simulink model "LACS"  (R2016b)
settings: Solver=VariableStepAuto  StartTime=0.0  StopTime=10  RelTol=1e-3
values from neighbouring files (symbols this model uses):
  coefficient = 0.8    [LACS.sldd]
  Detal_ref = 0.00022116955850615819 0.00022116955850615819 0.00024339323736781077 0.00026784369743330114 0.00029474273075037104 0.00032433393975435165 0.00035688482250496254 0.00039268904453642435 0.00043206891122917146 0.00047537805500027884 0.00052300435183202216 0.00057537308165349073 0.00063295034678974044 0.00069624676200566427 0.00076582142849131239 0.0008422862023284908 0.000926310265386283 0.0010186250    [LACS.sldd]    (also in path_generate.m = zeros(N,1))
  driver_decel = 4.0    [LACS.sldd]
  EgoLength = 3.048    [LACS.sldd]
  egopath = 0.0 0.25 0.5 0.75 1.0 1.25 1.5 1.7500000000000002 2.0 2.25 2.5 2.75 3.0 3.25 3.5000000000000004 3.75 4.0 4.25 4.5 4.75 5.0 5.25 5.5 5.75 6.0 6.25 6.5 6.75 7.0000000000000009 7.2499999999999991 7.5 7.75 8.0 8.25 8.5 8.75 9.0 9.25 9.5 9.75 10.0 10.25 10.5 10.75 11.0 11.25 11.5 11.75 12.0 12.25 12.5 12.75 13.0 13.25 13.5 13.750000000000002 14.000000000000002 14.250000000000002 14.499999999999998 14.7    [LACS.sldd]
  egoSpdLimit_H = 150.0    [LACS.sldd]
  egoSpdLimit_L = 10.0    [LACS.sldd]
  EgoWidth = 1.628    [LACS.sldd]
  ESA_Active = 3.0    [LACS.sldd]
  ESA_mask_1 = 31.0    [LACS.sldd]
  ESA_mask_2 = 15.0    [LACS.sldd]
  ESA_mask_3 = 255.0    [LACS.sldd]
  ESA_mask_4 = 31.0    [LACS.sldd]
  ESA_Passive = 1.0    [LACS.sldd]
  ESA_Standby = 2.0    [LACS.sldd]
  g = 9.8    [LACS.sldd]
  headwayoffset = 1.524    [LACS.sldd]
  LatAccelThershold = 0.05    [LACS.sldd]
  LatDis = 0.5    [LACS.sldd]
  LatSafetyThershold = 0.5    [LACS.sldd]
  LengthObj = 3.0    [LACS.sldd]
  ObjWidth = 2.0    [LACS.sldd]
  PB1_decel = 3.0    [LACS.sldd]
  PB2_decel = 5.0    [LACS.sldd]
  PB3_decel = 8.0    [LACS.sldd]
  Phi_dot_ref = 0.00085065224568106894 0.00085065224568106894 0.000936127966106986 0.0010301682404378703 0.0011336261186052523 0.0012474385378394444 0.001372634343205976 0.0015103430260158721 0.001661804233646022 0.0018283781058153412 0.0020115564932359636 0.0022129751145658549 0.0024344267064660809 0.0026778752189651235 0.0029454711038487576 0.0032395677369184911 0.0035627390050890382 0.0039177980756855638 0.004    [LACS.sldd]    (also in path_generate.m = zeros(N,1))
  Phi_ref = 0.00038406250525431664 0.00042271073336932769 0.00046524334565338114 0.00051204974395873044 0.000563558155980624 0.00062023946191088657 0.00068261138880285879 0.00075124310596315759 0.0008267602572639512 0.0009098504689462523 0.0010012693742370194 0.0011018471988988175 0.0012124959546271103 0.0013342172899504143 0.0014681110508986705 0.0016153846060911084 0.0017773629929370329 0.001955499943191484    [LACS.sldd]    (also in path_generate.m = phi_ref)
  SteerAngleLimit = 20.0    [LACS.sldd]
  SteerAngleSpdLimit = 20.0    [LACS.sldd]
  StrAngSpdThershold = 0.05    [LACS.sldd]
  StrAngThershold = 0.0    [LACS.sldd]
  Time2React = 1.2    [LACS.sldd]
  timeMargin = 0.5    [LACS.sldd]
  TTCthreshold1 = 2.5    [LACS.sldd]
  TTCthreshold3 = 1.0    [LACS.sldd]
  X_dot_ref = 10.0 10.0 10.0 9.9999999999999947 10.0 10.0 10.0 10.0 10.0 10.0 10.0 10.0 10.0 10.0 10.0 10.000000000000018 10.0 10.0 10.0 10.0 10.0 10.0 10.0 10.0 10.0 10.0 10.0 10.0 10.0 10.0 10.0 10.0 10.0 10.0 10.0 10.0 10.0 10.0 10.0 10.0 10.0 10.0 10.0 10.0 10.0 10.0 10.0 10.0 10.0 10.0 10.0 10.0 10.0 10.0 10.0 10.0 10.0 10.0 10.0 10.0 10.0 10.0 10.0 9.9999999999999289 10.0 10.0 10.0 10.0 10.0 10.0 10.0 10.    [LACS.sldd]    (also in path_generate.m = zeros(N,1))
  X_ref = 0.05 0.55 1.05 1.55 2.05 2.55 3.05 3.55 4.05 4.55 5.05 5.55 6.05 6.55 7.05 7.55 8.05 8.55 9.05 9.55 10.05 10.55 11.05 11.55 12.05 12.55 13.05 13.55 14.05 14.55 15.05 15.55 16.05 16.55 17.05 17.55 18.05 18.55 19.05 19.55 20.05 20.55 21.05 21.55 22.05 22.55 23.05 23.55 24.05 24.55 25.05 25.55 26.05 26.55 27.05 27.55 28.05 28.55 29.05 29.55 30.05 30.55 31.05 31.55 32.05 32.55 33.05 33.55 34.05 34.55    [LACS.sldd]    (also in path_generate.m = X_phi')
  Y_dot_ref = 0.0044363771042237217 0.0044363771042237217 0.00488273213335339 0.0053739322979981 0.0059144698111347933 0.0065092840662692251 0.0071638055584438178 0.0078840039934084845 0.0086764409570179273 0.0095483275445279979 0.01050758737719603 0.011562925461771293 0.012723903376023141 0.014001021290828194 0.015405807364013962 0.016950915064438028 0.018650229002128878 0.020518979854070446 0.0225738689793052    [LACS.sldd]    (also in path_generate.m = zeros(N,1))
  Y_ref = 0.0020016327462461514 0.0022031718511841521 0.0024249907063953382 0.0026691273130630077 0.0029378239279629127 0.0032335474185196523 0.0035590116218331136 0.0039172018997553045 0.0043114020994257287 0.0047452241472766251 0.005222640524503025 0.0057480198933628265 0.0063261661664513911 0.0069623613352525482 0.0076624123997939579 0.008432702767994656 0.0092802485212165574 0.010212759971323001 0.01123    [LACS.sldd]    (also in path_generate.m = zeros(N,1))
undefined symbols (not defined in the file or in its folder): ADR_ADRCycleTime, ADR_SteeringYawrateThresh_p, AEB_mask1, aubr, CAEB_AccelPdlPosLimit, CAEB_AccelPdlPosSpdThreshold, CAEB_CalAEBLongVelObjLimit_mps, CAEB_CalAEBVMaxDec_kmph, ESA_AESACTIVE, ESA_ERROR, ESA_ESAFunctionOFF, ESA_ESAFunctionON, ESA_ESASwichOFF, ESA_ESS_DriverSteeringNumThreshold, ESA_ESSACTIVE, ESA_ForewardCollissionLevel2, ESA_ForewardCollissionLevel3, ESA_OFF, ESA_PASSIVE, ESA_PLAN_AES, ESA_PLAN_ESSLEFT, ESA_PLAN_ESSRIGHT, ESA_PLAN_FAILURE, ESA_PLAN_OFF, ESA_PLAN_STANDBY, ESA_PLAN_WAIT, ESA_SPEEDLIMITH6_p, ESA_SPEEDLIMITH7_p, ESA_SPEEDLIMITL6_p, ESA_SPEEDLIMITL7_p, ESA_STANDBY, ESA_StrAngSpdT6_p, FromAngle2Rad, Kp, magnitude, tablebr, TTCthreshold, vubr
libraries: simulink x15, Solver_SF x9, simulink_extras x1
(part 4 of 5)

== system LACS/ESAsts/Passive2StandbyFlag/Subsystem3 ==
  flag : Inport
  Constant45 : Constant  Value=0  OutDataTypeStr=uint32
  Constant46 : Constant  OutDataTypeStr=uint32
  Multiport Switch7 : MultiPortSwitch  DataPortOrder=Zero-based contiguous  Inputs=2
  Shift Arithmetic : ArithShift  BitShiftNumberSource=Input port  BitShiftNumber=8  BitShiftDirection=Left
      settings: InputPortMap=u0,p1
  bitMask : Constant  Value=0  OutDataTypeStr=uint8
  maskCnst : Outport
  wires:
  flag/1 -> Multiport Switch7/1
  Multiport Switch7/1 -> maskCnst/1
  Constant46/1 -> Shift Arithmetic/1
  Constant45/1 -> Multiport Switch7/2
  Shift Arithmetic/1 -> Multiport Switch7/3
  bitMask/1 -> Shift Arithmetic/2

== system LACS/ESAsts/Passive2StandbyFlag/Subsystem4 ==
  flag : Inport
  Constant45 : Constant  Value=0  OutDataTypeStr=uint32
  Constant46 : Constant  OutDataTypeStr=uint32
  Multiport Switch7 : MultiPortSwitch  DataPortOrder=Zero-based contiguous  Inputs=2
  Shift Arithmetic : ArithShift  BitShiftNumberSource=Input port  BitShiftNumber=8  BitShiftDirection=Left
      settings: InputPortMap=u0,p1
  bitMask : Constant  Value=2  OutDataTypeStr=uint8
  maskCnst : Outport
  wires:
  flag/1 -> Multiport Switch7/1
  Multiport Switch7/1 -> maskCnst/1
  Constant46/1 -> Shift Arithmetic/1
  Constant45/1 -> Multiport Switch7/2
  Shift Arithmetic/1 -> Multiport Switch7/3
  bitMask/1 -> Shift Arithmetic/2

== system LACS/ESAsts/Passive2StandbyFlag/Subsystem5 ==
  flag : Inport
  Constant45 : Constant  Value=0  OutDataTypeStr=uint32
  Constant46 : Constant  OutDataTypeStr=uint32
  Multiport Switch7 : MultiPortSwitch  DataPortOrder=Zero-based contiguous  Inputs=2
  Shift Arithmetic : ArithShift  BitShiftNumberSource=Input port  BitShiftNumber=8  BitShiftDirection=Left
      settings: InputPortMap=u0,p1
  bitMask : Constant  Value=3  OutDataTypeStr=uint8
  maskCnst : Outport
  wires:
  flag/1 -> Multiport Switch7/1
  Multiport Switch7/1 -> maskCnst/1
  Constant46/1 -> Shift Arithmetic/1
  Constant45/1 -> Multiport Switch7/2
  Shift Arithmetic/1 -> Multiport Switch7/3
  bitMask/1 -> Shift Arithmetic/2

== system LACS/ESAsts/Passive2StandbyFlag1/LatAccelLimit ==
  Constant10 : Constant  Value=g
  Constant12 : Constant  Value=0.67
  Constant9 : Constant  Value=coefficient
  Divide : Product  Inputs=***
  Limit : Outport
  wires:
  Constant10/1 -> Divide/2
  Constant12/1 -> Divide/3
  Divide/1 -> Limit/1
  Constant9/1 -> Divide/1

== system LACS/ESAsts/Passive2StandbyFlag1/Subsystem1 ==
  flag : Inport
  Constant45 : Constant  Value=0  OutDataTypeStr=uint32
  Constant46 : Constant  OutDataTypeStr=uint32
  Multiport Switch7 : MultiPortSwitch  DataPortOrder=Zero-based contiguous  Inputs=2
  Shift Arithmetic : ArithShift  BitShiftNumberSource=Input port  BitShiftNumber=8  BitShiftDirection=Left
      settings: InputPortMap=u0,p1
  bitMask : Constant  Value=0  OutDataTypeStr=uint8
  maskCnst : Outport
  wires:
  flag/1 -> Multiport Switch7/1
  Multiport Switch7/1 -> maskCnst/1
  Constant46/1 -> Shift Arithmetic/1
  Constant45/1 -> Multiport Switch7/2
  Shift Arithmetic/1 -> Multiport Switch7/3
  bitMask/1 -> Shift Arithmetic/2

== system LACS/ESAsts/Passive2StandbyFlag1/Subsystem16 ==
  flag : Inport
  Constant45 : Constant  Value=0  OutDataTypeStr=uint32
  Constant46 : Constant  Value=2  OutDataTypeStr=uint32
  Multiport Switch7 : MultiPortSwitch  DataPortOrder=Zero-based contiguous  Inputs=2
  Shift Arithmetic : ArithShift  BitShiftNumberSource=Input port  BitShiftNumber=8  BitShiftDirection=Left
      settings: InputPortMap=u0,p1
  bitMask : Constant  Value=0  OutDataTypeStr=uint8
  maskCnst : Outport
  wires:
  flag/1 -> Multiport Switch7/1
  Multiport Switch7/1 -> maskCnst/1
  Constant46/1 -> Shift Arithmetic/1
  Constant45/1 -> Multiport Switch7/2
  Shift Arithmetic/1 -> Multiport Switch7/3
  bitMask/1 -> Shift Arithmetic/2

== system LACS/ESAsts/Passive2StandbyFlag1/Subsystem2 ==
  flag : Inport
  Constant45 : Constant  Value=0  OutDataTypeStr=uint32
  Constant46 : Constant  Value=3  OutDataTypeStr=uint32
  Multiport Switch7 : MultiPortSwitch  DataPortOrder=Zero-based contiguous  Inputs=2
  Shift Arithmetic : ArithShift  BitShiftNumberSource=Input port  BitShiftNumber=8  BitShiftDirection=Left
      settings: InputPortMap=u0,p1
  bitMask : Constant  Value=0  OutDataTypeStr=uint8
  maskCnst : Outport
  wires:
  bitMask/1 -> Shift Arithmetic/2
  Shift Arithmetic/1 -> Multiport Switch7/3
  Constant45/1 -> Multiport Switch7/2
  Constant46/1 -> Shift Arithmetic/1
  Multiport Switch7/1 -> maskCnst/1
  flag/1 -> Multiport Switch7/1

== system LACS/ESAsts/Passive2StandbyFlag1/Subsystem3 ==
  flag : Inport
  Constant45 : Constant  Value=0  OutDataTypeStr=uint32
  Constant46 : Constant  Value=4  OutDataTypeStr=uint32
  Multiport Switch7 : MultiPortSwitch  DataPortOrder=Zero-based contiguous  Inputs=2
  Shift Arithmetic : ArithShift  BitShiftNumberSource=Input port  BitShiftNumber=8  BitShiftDirection=Left
      settings: InputPortMap=u0,p1
  bitMask : Constant  Value=0  OutDataTypeStr=uint8
  maskCnst : Outport
  wires:
  bitMask/1 -> Shift Arithmetic/2
  Shift Arithmetic/1 -> Multiport Switch7/3
  Constant45/1 -> Multiport Switch7/2
  Constant46/1 -> Shift Arithmetic/1
  Multiport Switch7/1 -> maskCnst/1
  flag/1 -> Multiport Switch7/1

== system LACS/ESAsts/Passive2StandbyFlag1/Subsystem4 ==
  flag : Inport
  Constant45 : Constant  Value=0  OutDataTypeStr=uint32
  Constant46 : Constant  Value=5  OutDataTypeStr=uint32
  Multiport Switch7 : MultiPortSwitch  DataPortOrder=Zero-based contiguous  Inputs=2
  Shift Arithmetic : ArithShift  BitShiftNumberSource=Input port  BitShiftNumber=8  BitShiftDirection=Left
      settings: InputPortMap=u0,p1
  bitMask : Constant  Value=0  OutDataTypeStr=uint8
  maskCnst : Outport
  wires:
  flag/1 -> Multiport Switch7/1
  Multiport Switch7/1 -> maskCnst/1
  Constant46/1 -> Shift Arithmetic/1
  Constant45/1 -> Multiport Switch7/2
  Shift Arithmetic/1 -> Multiport Switch7/3
  bitMask/1 -> Shift Arithmetic/2

== system LACS/ESAsts/Passive2StandbyFlag1/Subsystem5 ==
  flag : Inport
  Constant45 : Constant  Value=0  OutDataTypeStr=uint32
  Constant46 : Constant  Value=6  OutDataTypeStr=uint32
  Multiport Switch7 : MultiPortSwitch  DataPortOrder=Zero-based contiguous  Inputs=2
  Shift Arithmetic : ArithShift  BitShiftNumberSource=Input port  BitShiftNumber=8  BitShiftDirection=Left
      settings: InputPortMap=u0,p1
  bitMask : Constant  Value=0  OutDataTypeStr=uint8
  maskCnst : Outport
  wires:
  flag/1 -> Multiport Switch7/1
  Multiport Switch7/1 -> maskCnst/1
  Constant46/1 -> Shift Arithmetic/1
  Constant45/1 -> Multiport Switch7/2
  Shift Arithmetic/1 -> Multiport Switch7/3
  bitMask/1 -> Shift Arithmetic/2

== system LACS/ESAsts/Stanby2PassiveFlag/LatAccelLimit ==
  Constant10 : Constant  Value=g
  Constant12 : Constant  Value=0.67
  Constant9 : Constant  Value=coefficient
  Divide : Product  Inputs=***
  Limit : Outport
  wires:
  Constant10/1 -> Divide/2
  Constant12/1 -> Divide/3
  Divide/1 -> Limit/1
  Constant9/1 -> Divide/1

== system LACS/ESAsts/Stanby2PassiveFlag/Subsystem1 ==
  flag : Inport
  Constant45 : Constant  Value=0  OutDataTypeStr=uint32
  Constant46 : Constant  OutDataTypeStr=uint32
  Multiport Switch7 : MultiPortSwitch  DataPortOrder=Zero-based contiguous  Inputs=2
  Shift Arithmetic : ArithShift  BitShiftNumberSource=Input port  BitShiftNumber=8  BitShiftDirection=Left
      settings: InputPortMap=u0,p1
  bitMask : Constant  Value=3  OutDataTypeStr=uint8
  maskCnst : Outport
  wires:
  flag/1 -> Multiport Switch7/1
  Multiport Switch7/1 -> maskCnst/1
  Constant46/1 -> Shift Arithmetic/1
  Constant45/1 -> Multiport Switch7/2
  Shift Arithmetic/1 -> Multiport Switch7/3
  bitMask/1 -> Shift Arithmetic/2

== system LACS/ESAsts/Stanby2PassiveFlag/Subsystem3 ==
  flag : Inport
  Constant45 : Constant  Value=0  OutDataTypeStr=uint32
  Constant46 : Constant  OutDataTypeStr=uint32
  Multiport Switch7 : MultiPortSwitch  DataPortOrder=Zero-based contiguous  Inputs=2
  Shift Arithmetic : ArithShift  BitShiftNumberSource=Input port  BitShiftNumber=8  BitShiftDirection=Left
      settings: InputPortMap=u0,p1
  bitMask : Constant  Value=0  OutDataTypeStr=uint8
  maskCnst : Outport
  wires:
  flag/1 -> Multiport Switch7/1
  Multiport Switch7/1 -> maskCnst/1
  Constant46/1 -> Shift Arithmetic/1
  Constant45/1 -> Multiport Switch7/2
  Shift Arithmetic/1 -> Multiport Switch7/3
  bitMask/1 -> Shift Arithmetic/2

== system LACS/ESAsts/Stanby2PassiveFlag/Subsystem4 ==
  flag : Inport
  Constant45 : Constant  Value=0  OutDataTypeStr=uint32
  Constant46 : Constant  OutDataTypeStr=uint32
  Multiport Switch7 : MultiPortSwitch  DataPortOrder=Zero-based contiguous  Inputs=2
  Shift Arithmetic : ArithShift  BitShiftNumberSource=Input port  BitShiftNumber=8  BitShiftDirection=Left
      settings: InputPortMap=u0,p1
  bitMask : Constant  OutDataTypeStr=uint8
  maskCnst : Outport
  wires:
  flag/1 -> Multiport Switch7/1
  Multiport Switch7/1 -> maskCnst/1
  Constant46/1 -> Shift Arithmetic/1
  Constant45/1 -> Multiport Switch7/2
  Shift Arithmetic/1 -> Multiport Switch7/3
  bitMask/1 -> Shift Arithmetic/2

== system LACS/ESAsts/Stanby2PassiveFlag/Subsystem5 ==
  flag : Inport
  Constant45 : Constant  Value=0  OutDataTypeStr=uint32
  Constant46 : Constant  OutDataTypeStr=uint32
  Multiport Switch7 : MultiPortSwitch  DataPortOrder=Zero-based contiguous  Inputs=2
  Shift Arithmetic : ArithShift  BitShiftNumberSource=Input port  BitShiftNumber=8  BitShiftDirection=Left
      settings: InputPortMap=u0,p1
  bitMask : Constant  Value=2  OutDataTypeStr=uint8
  maskCnst : Outport
  wires:
  flag/1 -> Multiport Switch7/1
  Multiport Switch7/1 -> maskCnst/1
  Constant46/1 -> Shift Arithmetic/1
  Constant45/1 -> Multiport Switch7/2
  Shift Arithmetic/1 -> Multiport Switch7/3
  bitMask/1 -> Shift Arithmetic/2

== system LACS/ESAsts/Standby to Active/LatAccelLimit ==
  Constant10 : Constant  Value=g
  Constant12 : Constant  Value=0.67
  Constant9 : Constant  Value=coefficient
  Divide : Product  Inputs=***
  Limit : Outport
  wires:
  Constant10/1 -> Divide/2
  Constant12/1 -> Divide/3
  Divide/1 -> Limit/1
  Constant9/1 -> Divide/1

== system LACS/ESAsts/Standby to Active/Subsystem1 ==
  flag : Inport
  Constant45 : Constant  Value=0  OutDataTypeStr=uint32
  Constant46 : Constant  OutDataTypeStr=uint32
  Multiport Switch7 : MultiPortSwitch  DataPortOrder=Zero-based contiguous  Inputs=2
  Shift Arithmetic : ArithShift  BitShiftNumberSource=Input port  BitShiftNumber=8  BitShiftDirection=Left
      settings: InputPortMap=u0,p1
  bitMask : Constant  OutDataTypeStr=uint8
  maskCnst : Outport
  wires:
  flag/1 -> Multiport Switch7/1
  Multiport Switch7/1 -> maskCnst/1
  Constant46/1 -> Shift Arithmetic/1
  Constant45/1 -> Multiport Switch7/2
  Shift Arithmetic/1 -> Multiport Switch7/3
  bitMask/1 -> Shift Arithmetic/2

== system LACS/ESAsts/Standby to Active/Subsystem16 ==
  flag : Inport
  Constant45 : Constant  Value=0  OutDataTypeStr=uint32
  Constant46 : Constant  OutDataTypeStr=uint32
  Multiport Switch7 : MultiPortSwitch  DataPortOrder=Zero-based contiguous  Inputs=2
  Shift Arithmetic : ArithShift  BitShiftNumberSource=Input port  BitShiftNumber=8  BitShiftDirection=Left
      settings: InputPortMap=u0,p1
  bitMask : Constant  Value=2  OutDataTypeStr=uint8
  maskCnst : Outport
  wires:
  flag/1 -> Multiport Switch7/1
  Multiport Switch7/1 -> maskCnst/1
  Constant46/1 -> Shift Arithmetic/1
  Constant45/1 -> Multiport Switch7/2
  Shift Arithmetic/1 -> Multiport Switch7/3
  bitMask/1 -> Shift Arithmetic/2

== system LACS/ESAsts/Standby to Active/Subsystem2 ==
  flag : Inport
  Constant45 : Constant  Value=0  OutDataTypeStr=uint32
  Constant46 : Constant  OutDataTypeStr=uint32
  Multiport Switch7 : MultiPortSwitch  DataPortOrder=Zero-based contiguous  Inputs=2
  Shift Arithmetic : ArithShift  BitShiftNumberSource=Input port  BitShiftNumber=8  BitShiftDirection=Left
      settings: InputPortMap=u0,p1
  bitMask : Constant  Value=3  OutDataTypeStr=uint8
  maskCnst : Outport
  wires:
  bitMask/1 -> Shift Arithmetic/2
  Shift Arithmetic/1 -> Multiport Switch7/3
  Constant45/1 -> Multiport Switch7/2
  Constant46/1 -> Shift Arithmetic/1
  Multiport Switch7/1 -> maskCnst/1
  flag/1 -> Multiport Switch7/1

== system LACS/ESAsts/Standby to Active/Subsystem3 ==
  flag : Inport
  Constant45 : Constant  Value=0  OutDataTypeStr=uint32
  Constant46 : Constant  OutDataTypeStr=uint32
  Multiport Switch7 : MultiPortSwitch  DataPortOrder=Zero-based contiguous  Inputs=2
  Shift Arithmetic : ArithShift  BitShiftNumberSource=Input port  BitShiftNumber=8  BitShiftDirection=Left
      settings: InputPortMap=u0,p1
  bitMask : Constant  Value=4  OutDataTypeStr=uint8
  maskCnst : Outport
  wires:
  bitMask/1 -> Shift Arithmetic/2
  Shift Arithmetic/1 -> Multiport Switch7/3
  Constant45/1 -> Multiport Switch7/2
  Constant46/1 -> Shift Arithmetic/1
  Multiport Switch7/1 -> maskCnst/1
  flag/1 -> Multiport Switch7/1

== system LACS/ESAsts/Standby to Active/Subsystem4 ==
  flag : Inport
  Constant45 : Constant  Value=0  OutDataTypeStr=uint32
  Constant46 : Constant  OutDataTypeStr=uint32
  Multiport Switch7 : MultiPortSwitch  DataPortOrder=Zero-based contiguous  Inputs=2
  Shift Arithmetic : ArithShift  BitShiftNumberSource=Input port  BitShiftNumber=8  BitShiftDirection=Left
      settings: InputPortMap=u0,p1
  bitMask : Constant  Value=5  OutDataTypeStr=uint8
  maskCnst : Outport
  wires:
  flag/1 -> Multiport Switch7/1
  Multiport Switch7/1 -> maskCnst/1
  Constant46/1 -> Shift Arithmetic/1
  Constant45/1 -> Multiport Switch7/2
  Shift Arithmetic/1 -> Multiport Switch7/3
  bitMask/1 -> Shift Arithmetic/2

== system LACS/ESAsts/Standby to Active/Subsystem5 ==
  flag : Inport
  Constant45 : Constant  Value=0  OutDataTypeStr=uint32
  Constant46 : Constant  OutDataTypeStr=uint32
  Multiport Switch7 : MultiPortSwitch  DataPortOrder=Zero-based contiguous  Inputs=2
  Shift Arithmetic : ArithShift  BitShiftNumberSource=Input port  BitShiftNumber=8  BitShiftDirection=Left
      settings: InputPortMap=u0,p1
  bitMask : Constant  Value=6  OutDataTypeStr=uint8
  maskCnst : Outport
  wires:
  flag/1 -> Multiport Switch7/1
  Multiport Switch7/1 -> maskCnst/1
  Constant46/1 -> Shift Arithmetic/1
  Constant45/1 -> Multiport Switch7/2
  Shift Arithmetic/1 -> Multiport Switch7/3
  bitMask/1 -> Shift Arithmetic/2

== system LACS/ESAsts/Standby to Active/Subsystem6 ==
  flag : Inport
  Constant45 : Constant  Value=0  OutDataTypeStr=uint32
  Constant46 : Constant  OutDataTypeStr=uint32
  Multiport Switch7 : MultiPortSwitch  DataPortOrder=Zero-based contiguous  Inputs=2
  Shift Arithmetic : ArithShift  BitShiftNumberSource=Input port  BitShiftNumber=8  BitShiftDirection=Left
      settings: InputPortMap=u0,p1
  bitMask : Constant  Value=0  OutDataTypeStr=uint8
  maskCnst : Outport
  wires:
  flag/1 -> Multiport Switch7/1
  Multiport Switch7/1 -> maskCnst/1
  Constant46/1 -> Shift Arithmetic/1
  Constant45/1 -> Multiport Switch7/2
  Shift Arithmetic/1 -> Multiport Switch7/3
  bitMask/1 -> Shift Arithmetic/2

== system LACS/ESAsts/Standby to Active/Subsystem7 ==
  flag : Inport
  Constant45 : Constant  Value=0  OutDataTypeStr=uint32
  Constant46 : Constant  OutDataTypeStr=uint32
  Multiport Switch7 : MultiPortSwitch  DataPortOrder=Zero-based contiguous  Inputs=2
  Shift Arithmetic : ArithShift  BitShiftNumberSource=Input port  BitShiftNumber=8  BitShiftDirection=Left
      settings: InputPortMap=u0,p1
  bitMask : Constant  Value=7  OutDataTypeStr=uint8
  maskCnst : Outport
  wires:
  flag/1 -> Multiport Switch7/1
  Multiport Switch7/1 -> maskCnst/1
  Constant46/1 -> Shift Arithmetic/1
  Constant45/1 -> Multiport Switch7/2
  Shift Arithmetic/1 -> Multiport Switch7/3
  bitMask/1 -> Shift Arithmetic/2

== stateflow chart LACS/ESAManager ==
  state ON
    FuncStsReq = ESA_ESAFunctionON;
    state STANDBY
      en, du:
      EsaSts = ESA_STANDBY;
      EsaSts_plan = ESA_PLAN_WAIT;
      TakeoverFbk = false;
    state PASSIVE
      en, du:
      EsaSts = ESA_PASSIVE;
      EsaSts_plan = ESA_PLAN_STANDBY;
      TakeoverFbk = false;
    state ACTIVE
      TakeoverFbk = true;
      state ESSACTIVE
        en, du:
        EsaSts = ESA_ESSACTIVE;
        state ESSRIGHT
          en, du:
          EsaSts_plan = ESA_PLAN_ESSRIGHT;
        state ESSLEFT
          en, du:
          EsaSts_plan = ESA_PLAN_ESSLEFT;
      state ASSACTIVE
        en, du:
        EsaSts = ESA_AESACTIVE;
        EsaSts_plan = ESA_PLAN_AES;
    (default) -> PASSIVE
    PASSIVE -> STANDBY : /*C4*/
        | after(1, tick)
        | [fc4]
    STANDBY -> PASSIVE [order 3] : /*C5*/
        | after(1, tick)
        | [fc5]
    ACTIVE -> PASSIVE : /*C8*/
        | after(1, tick)
        | [fc8]
    STANDBY -> ESSLEFT [order 1] : /*C6*/
        | after(1, tick)
        | [fc6_left]
    STANDBY -> ESSRIGHT [order 4] : after(1, tick)
        | [fc6_right]
    STANDBY -> ASSACTIVE [order 2] : /*C7*/
        | after(1, tick)
        | [fc7]
  state OFF
    en, du:
    EsaSts = ESA_OFF;
    EsaSts_plan = ESA_PLAN_OFF;
    TakeoverFbk = false;
    FuncStsReq = ESA_ESAFunctionOFF;
  state ERROR
    en, du:
    EsaSts = ESA_ERROR;
    EsaSts_plan = ESA_PLAN_FAILURE;
    TakeoverFbk = false;
    FuncStsReq = ESA_ESAFunctionOFF;
  (default) -> ON
  OFF -> ON : /**C1*/
      | after(1, tick)
      | [fc1]
  ON -> OFF [order 1] : /*C2**/
      | after(1, tick)
      | [fc2]
  ERROR -> ON : /*C10*/
      | after(1, tick)
      | [fc10]
  ON -> ERROR [order 2] : /*C9*/
      | after(1, tick)
      | [fc9]
  data: fc1 input boolean; fc2 input boolean; ESA_AESACTIVE parameter uint8; ESA_ERROR parameter uint8; ESA_ESSACTIVE parameter uint8; ESA_OFF parameter uint8; ESA_PASSIVE parameter uint8; ESA_STANDBY parameter uint8; EsaSts output uint8; fc4 input boolean; fc5 input boolean; fc6_left input boolean; fc6_right input boolean; fc7 input boolean; fc8 input boolean; fc9 input boolean; fc10 input boolean; FuncStsReq output uint8; TakeoverFbk output boolean; EsaSts_plan output uint8; ESA_PLAN_AES parameter; ESA_PLAN_ESSLEFT parameter; ESA_PLAN_ESSRIGHT parameter; ESA_PLAN_FAILURE parameter; ESA_PLAN_OFF parameter; ESA_PLAN_STANDBY parameter; ESA_PLAN_WAIT parameter; ESA_ESAFunctionOFF parameter uint8; ESA_ESAFunctionON parameter uint8

== stateflow chart LACS/AEB_System/Chart ==
  state default_state
    entry:CMpa = 0;
    Alart = 0;
    Break_signal = 0;
  state Init_1_state1
    du:
    if(30<Distance<40)
    CMpa = 2;
    Alart = 1;
    Break_signal = 1;
    elseif(20<Distance<30)
    CMpa = 5;
    Alart = 2;
    Break_signal = 1;
    elseif(10<Distance<20)
    CMpa = 8;
    Alart = 3;
    Break_signal = 1;
    end
  (default) -> default_state
  default_state -> Init_1_state1 : [Distance<=40]
  Init_1_state1 -> default_state : [Distance>40]
  data: Distance input; V_difference input; V_Speed input; CMpa output; Alart output; Break_signal output

== stateflow chart LACS/AEB//ESA Comprehensive Decision ==
  note: AEB/ESA共同决策逻辑
  state System_Active
    state ModeSwitch
    state ESA_ON
      state Standby
      state Passive
      state Active
        state AES
        state ESS
          state ESS_Right
          state ESS_Left
      System_Active.ESA_ON.Passive -> System_Active.ESA_ON.Standby
      System_Active.ESA_ON.Standby -> System_Active.ESA_ON.Passive [order 4]
      System_Active.ESA_ON.Active -> System_Active.ESA_ON.Passive
      System_Active.ESA_ON.Standby -> ESS_Left [order 2]
      System_Active.ESA_ON.Standby -> ESS_Right [order 3]
      System_Active.ESA_ON.Standby -> AES [order 1]
    state AEB_ON
      state Standby
      state Passive
      state Active
        state CCR
        state VRU
      System_Active.AEB_ON.Passive -> System_Active.AEB_ON.Standby
      System_Active.AEB_ON.Standby -> System_Active.AEB_ON.Passive [order 3]
      System_Active.AEB_ON.Active -> System_Active.AEB_ON.Passive
      System_Active.AEB_ON.Standby -> CCR [order 1]
      System_Active.AEB_ON.Standby -> VRU [order 2]
    (default) -> ModeSwitch
    ModeSwitch -> AEB_ON [order 1] : [AEBCrashAvoid==1&&ESATakeOverReq==0]
    ModeSwitch -> ESA_ON [order 2] : [AEBCrashAvoid==0&&ESATakeOverReq==1]
  state OFF
  (default) -> System_Active
  OFF -> System_Active
  System_Active -> OFF

== matlab function LACS/Subsystem/err_kappa_calculate_module ==
  data: x input; kr output; y input; phi input; vx input; vy input; phi_dot input; xr input; yr input; thetar input; kappar input; err output
function [kr,err] = fcn(x,y,phi,vx,vy,phi_dot,xr,yr,thetar,kappar)
    n=length(xr);
    d_min=(x-xr(1))^2+(y-yr(1))^2;
    min=1;
    for i=1:n
        d=(x-xr(i))^2+(y-yr(i))^2;
        if d<d_min
            d_min=d;
            min=i;
        end
    end
    dmin=min;
    tor=[cos(thetar(dmin));sin(thetar(dmin))];
    nor=[-sin(thetar(dmin));cos(thetar(dmin))];
    d_err=[x-xr(dmin);y-yr(dmin)];
    ed=nor'*d_err;
    es=tor'*d_err;
    %projection_point_thetar=thetar(dmin);%apollo
    projection_point_thetar=thetar(dmin)+kappar(dmin)*es;
    ed_dot=vy*cos(phi-projection_point_thetar)+vx*sin(phi-projection_point_thetar);
    %%%%%%%%%
    ephi=sin(phi-projection_point_thetar);
    %%%%%%%%%
    s_dot=vx*cos(phi-projection_point_thetar)-vy*sin(phi-projection_point_thetar);
    s_dot=s_dot/(1-kappar(dmin)*ed);
    ephi_dot=phi_dot-kappar(dmin)*s_dot;
    kr=kappar(dmin);
    err=[ed;ed_dot;ephi;ephi_dot];
    
    
    
    
    
    
    
    
    
    
    
    


end

== matlab function LACS/Subsystem/forword_control ==
  data: vx input; a input; forword_angle output; b input; m input; cf input; cr input; k input; kr input
function forword_angle = fcn(vx,a,b,m,cf,cr,k,kr)
    forword_angle=kr*(a+b-b*k(3)-(m*vx*vx/(a+b))*((b/cf)+(a/cr)*k(3)-(a/cr)));
end

== matlab function LACS/Subsystem/last_angle ==
  data: k input; angle output; err input; forword_angle input
function angle = fcn(k,err,forword_angle)

    angle=-k*err+forword_angle;
end

== matlab function LACS/Subsystem/lqr_offline ==
  data: k1 input; k output; k2 input; k3 input; k4 input; vx input
function k  = fcn(k1,k2,k3,k4,vx)
    if abs(vx)<0.01
        k=[0,0,0,0];
    else
        index=round(vx/0.01);
        k=[k1(index),k2(index),k3(index),k4(index)];
    end
end

== matlab function LACS/Subsystem/predict_module ==
  data: x input; pre_x output; y input; phi input; vx input; vy input; phi_dot input; ts input; pre_y output; pre_phi output; pre_vx output; pre_vy output; pre_phi_dot output
function [pre_x,pre_y,pre_phi,pre_vx,pre_vy,pre_phi_dot] = fcn(x,y,phi,vx,vy,phi_dot,ts)
    pre_x=x+vx*ts*cos(phi)-vy*ts*sin(phi);
    pre_y=y+vy*ts*cos(phi)+vx*ts*sin(phi);
    pre_phi=phi+phi_dot*ts;
    pre_vx=vx;
    pre_vy=vy;
    pre_phi_dot=phi_dot;
end

== matlab function LACS/LQR/err_kappa_calculate_module ==
  data: x input; kr output; y input; phi input; vx input; vy input; phi_dot input; xr input; yr input; thetar input; kappar input; err output; es output; s_dot output
function [kr,err,es,s_dot] = fcn(x,y,phi,vx,vy,phi_dot,xr,yr,thetar,kappar)
    
    tor=[cos(thetar);sin(thetar)];
    nor=[-sin(thetar);cos(thetar)];
    d_err=[x-xr;y-yr];
    ed=nor'*d_err;
    es=tor'*d_err;
    %projection_point_thetar=thetar(dmin);%apollo
    projection_point_thetar=thetar+kappar*es;
    ed_dot=vy*cos(phi-projection_point_thetar)+vx*sin(phi-projection_point_thetar);
    %%%%%%%%%
    ephi=sin(phi-projection_point_thetar);
    %%%%%%%%%
    ss_dot=vx*cos(phi-projection_point_thetar)-vy*sin(phi-projection_point_thetar);
    s_dot=ss_dot/(1-kappar*ed);
    ephi_dot=phi_dot-kappar*s_dot;
    kr=kappar;
    err=[ed;ed_dot;ephi;ephi_dot];
    
    
    
    
    
    
    
    
    
    
    
    


end

== matlab function LACS/LQR/forword_control ==
  data: vx input; a input; forword_angle output; b input; m input; cf input; cr input; k input; kr input
function forword_angle = fcn(vx,a,b,m,cf,cr,k,kr)
    forword_angle=kr*(a+b-b*k(3)-(m*vx*vx/(a+b))*((b/cf)+(a/cr)*k(3)-(a/cr)));
end

== matlab function LACS/LQR/last_angle ==
  data: k input; angle output; err input; forword_angle input
function angle = fcn(k,err,forword_angle)

    angle=-k*err+forword_angle;
end

== matlab function LACS/LQR/lqr_offline ==
  data: k1 input; k output; k2 input; k3 input; k4 input; vx input
function k  = fcn(k1,k2,k3,k4,vx)
    if abs(vx)<0.01
        k=[0,0,0,0];
    else
        index=round(vx/0.01);
        k=[k1(index),k2(index),k3(index),k4(index)];
    end
end

== matlab function LACS/LQR/predict_module ==
  data: x input; pre_x output; y input; phi input; vx input; vy input; phi_dot input; ts input; pre_y output; pre_phi output; pre_vx output; pre_vy output; pre_phi_dot output
function [pre_x,pre_y,pre_phi,pre_vx,pre_vy,pre_phi_dot] = fcn(x,y,phi,vx,vy,phi_dot,ts)
    pre_x=x+vx*ts*cos(phi)-vy*ts*sin(phi);
    pre_y=y+vy*ts*cos(phi)+vx*ts*sin(phi);
    pre_phi=phi+phi_dot*ts;
    pre_vx=vx;
    pre_vy=vy;
    pre_phi_dot=phi_dot;
end

== matlab function LACS/MATLAB Function ==
  data: vx input; v output; vy input
function v = fcn(vx,vy)
    v=sqrt(vx^2+vy^2);

== matlab function LACS/double_pid_controller/MATLAB Function1 ==
  data: x input; thr output; brake output
function [thr,brake] = fcn(x)
    %正数代表油门，负数代表刹车
    %不允许同时踩油门和刹车
    if x>=0
        thr=x;
        brake=0;
    else
        thr=0;
        brake=-x;
    end

== matlab function LACS/double_pid_controller/moto model ==
  data: thr input; torque output; rpm input
function torque = fcn(thr,rpm)
Tmax=380*thr;
    if (rpm<=4523)
        torque=Tmax;
    else
        torque=Tmax*4523/rpm;
    end
end

== matlab function LACS/planning ==
  data: vp output; ap output; t input; xr output; yr output; thetar output; kr output
function [vp,ap,xr,yr,thetar,kr] = fcn(t)
    dx=100; %向前移动100m，向左移动20m，运动时间30s
    dy=10;
    T=30;
    xstart=[0,0,0]; %起点和终点的位置，速度，加速度
    xend=[dx,0,0];
    ystart=[0,0,0];
    yend=[dy,0,0];
    a=zeros(1,6);   %五次多项式有六个系数
    b=zeros(1,6);
    
    %纵向的五次多项式系数
    a(1)=xstart(1);
    a(2)=xstart(2);
    a(3)=xstart(3)/2;
    %求解a(4),a(5),a(6)
    A1=[T^3,T^4,T^5;
        3*T^2,4*T^3,5*T^4;
        6*T,12*T^2,20*T^3];
    B1=[xend(1)-a(1)-a(2)*T-a(3)*T^2;
        xend(2)-a(2)-2*a(3)*T;
        xend(3)-2*a(3)];
    xs=inv(A1)*B1;
    a(4)=xs(1);
    a(5)=xs(2);
    a(6)=xs(3);
    %横向的五次多项式系数
    b(1)=ystart(1);
    b(2)=ystart(2);
    b(3)=ystart(3)/2;
    A2=[dx^3,dx^4,dx^5;
        3*dx^2,4*dx^3,5*dx^4;
        6*dx,12*dx^2,20*dx^3];
    B2=[yend(1)-b(1)-b(2)*dx-b(3)*dx^2;
        yend(2)-b(2)-2*b(3)*dx;
        yend(3)-2*b(3)];
    ys=inv(A2)*B2;
    b(4)=ys(1);
    b(5)=ys(2);
    b(6)=ys(3);
    
    %求解规划轨迹的位置，速度，加速度，曲率
    xr=a(1)+a(2)*t+a(3)*t^2+a(4)*t^3+a(5)*t^4+a(6)*t^5;
    yr=b(1)+b(2)*xr+b(3)*xr^2+b(4)*xr^3+b(5)*xr^4+b(6)*xr^5;
    
    xr_dot=a(2)+2*a(3)*t+3*a(4)*t^2+4*a(5)*t^3+5*a(6)*t^4;
    yr_dx=b(2)+2*b(3)*xr+3*b(4)*xr^2+4*b(5)*xr^3+5*b(6)*xr^4;
    yr_dot=yr_dx*xr_dot;
    
    thetar=atan(yr_dx);
    
    xr_dot2=2*a(3)+6*a(4)*t+12*a(5)*t^2+20*a(6)*t^3;
    yr_dx2=2*b(3)+6*b(4)*xr+12*b(5)*xr^2+20*b(6)*xr^3;
    yr_dot2=yr_dx2*xr_dot^2+yr_dx*xr_dot2;
    
    kr=yr_dx2/((1+yr_dx^2)^1.5);    %曲率
    
    vp=sqrt(xr_dot^2+yr_dot^2);
    
    if xr_dot2>=0
        ap=sqrt(xr_dot2^2+yr_dot2^2);
    else
        ap=-sqrt(xr_dot2^2+yr_dot2^2);
    end

== stateflow chart LACS/PassengerAEBManagement ==
  note: [(AEBSwitch_flag==0)&&(VehicleSpeed_kmph<4)]
  state On
    state Active
      state Vehicle
        en:
        PasgerAEBReq_flag=1;
        PasgerAEBState_enum=3;
        PasgerAEBTarObjType=2;
        du:
        AEBVLastTimeCLK=AEBVLastTimeCLK+1;
        ex:
        AEBVLastTimeCLK=1;
      state Pedestrain
        state P1
          en:
          PasgerAEBReq_flag=1;
          PasgerAEBState_enum=3;
          PasgerAEBTarObjType=1;
          du:
          AEBP1LastTimeCLK=AEBP1LastTimeCLK+1;
          ex:
          AEBP1LastTimeCLK=1;
        state P2
          en:
          PasgerAEBReq_flag=1;
          PasgerAEBState_enum=3;
          PasgerAEBTarObjType=1;
          du:
          AEBP2LastTimeCLK=AEBP2LastTimeCLK+1;
          ex:
          AEBP2LastTimeCLK=1;
      (default) -> Vehicle
    state Passive
      en:
      PasgerAEBReq_flag=0;
      PasgerAEBState_enum=1;
      PasgerAEBTarObjType=0;
    state Standby
      en:
      PasgerAEBReq_flag=0;
      PasgerAEBState_enum=2;
      PasgerAEBTarObjType=0;
    (default) -> Passive
    Active -> Passive : [(AEBActiveToPassive_flag==1)||(AEBVLastTimeCLK>=(CalAEBLastTime_s/CyclicTime_s))||(AEBP1LastTimeCLK>=(CalAEBLastTime_s/CyclicTime_s))...
        | ||(AEBP2LastTimeCLK>=(CalAEBLastTime_s/CyclicTime_s))]
    Passive -> Standby : [AEBPassiveToStandby_flag==1]
    Standby -> Passive [order 1] : [AEBStandbyToPassive_flag==1]
    Standby -> Vehicle [order 2] : [AEBVStandbyToActive_Flag==1]
    Standby -> P1 [order 4] : [AEBP1StandbyToActive_Flag==1]
    Standby -> P2 [order 3] : [AEBP2StandbyToActive_Flag==1]
  state Off
    en:
    PasgerAEBReq_flag=0;
    PasgerAEBState_enum=0;
    PasgerAEBTarObjType=0;
  state Initial
  state Failure
    en:
    PasgerAEBReq_flag=0;
    PasgerAEBState_enum=4;
    PasgerAEBTarObjType=0;
  note: 
  On -> Off [order 1] : [(AEBSwitch_flag==0)]
  Off -> Passive : [(AEBSwitch_flag==1)&&(AebFcwConstraintCondition==0)]
  Failure -> Off [order 2] : [(AEBSwitch_flag==0)]
  (default) -> Initial
  Failure -> On [order 1] : [(AEBSwitch_flag==1)&&(AebFcwConstraintCondition==0)]
  Initial -> Failure [order 1] : [AebFcwConstraintCondition>0]
  On -> Failure [order 2] : [(AEBSwitch_flag==1)&&(AebFcwConstraintCondition>0)]
  Initial -> On [order 2] : [AebFcwConstraintCondition==0]
  data: AEBFuncConfigEnable_flag input; AEBPassiveToStandby_flag input; AEBActiveToPassive_flag input; AEBVStandbyToActive_Flag input; AEBStandbyToPassive_flag input; AEBP1StandbyToActive_Flag input; AEBP2StandbyToActive_Flag input; AEBError_flag input boolean; AEBSwitch_flag input; PasgerAEBReq_flag output uint8; PasgerAEBState_enum output uint8; PasgerAEBTarObjType output uint8; VehicleSpeed_kmph input; AebFcwConstraintCondition input; CyclicTime_s input; CalAEBLastTime_s input; AEBVLastTimeCLK local double; AEBP1LastTimeCLK local double; AEBP2LastTimeCLK local double
  data AEBFuncConfigEnable_flag settings: description=$TL$ date=20191130T134642; inheritscaling=1; $TL$
  data AEBPassiveToStandby_flag settings: description=$TL$ date=20191130T134646; inheritscaling=1; $TL$
  data AEBVStandbyToActive_Flag settings: description=$TL$ date=20191130T134649; inheritscaling=1; $TL$
  data AEBP1StandbyToActive_Flag settings: description=$TL$ date=20191130T134653; inheritscaling=1; $TL$
  data AEBSwitch_flag settings: description=$TL$ date=20191130T134638; inheritscaling=1; $TL$
  data AebFcwConstraintCondition settings: description=$TL$ date=20191130T134638; inheritscaling=1; $TL$

== stateflow chart LACS/AEB//ESA Comprehensive Decision1 ==
  note: AEB/ESA共同决策逻辑
  state System_Active
    state ModeSwitch
    state ESA_ON
      state Standby
      state Passive
      state Active
        state AES
        state ESS
          state ESS_Right
          state ESS_Left
      System_Active.ESA_ON.Passive -> System_Active.ESA_ON.Standby
      System_Active.ESA_ON.Standby -> System_Active.ESA_ON.Passive [order 4]
      System_Active.ESA_ON.Active -> System_Active.ESA_ON.Passive
      System_Active.ESA_ON.Standby -> ESS_Left [order 2]
      System_Active.ESA_ON.Standby -> ESS_Right [order 3]
      System_Active.ESA_ON.Standby -> AES [order 1]
    state AEB_ON
      state Standby
      state Passive
      state Active
        state CCR
        state VRU
      System_Active.AEB_ON.Passive -> System_Active.AEB_ON.Standby
      System_Active.AEB_ON.Standby -> System_Active.AEB_ON.Passive [order 3]
      System_Active.AEB_ON.Active -> System_Active.AEB_ON.Passive
      System_Active.AEB_ON.Standby -> CCR [order 1]
      System_Active.AEB_ON.Standby -> VRU [order 2]
    (default) -> ModeSwitch
    ModeSwitch -> AEB_ON [order 1] : [AEBCrashAvoid==1&&ESATakeOverReq==0]
    ModeSwitch -> ESA_ON [order 2] : [AEBCrashAvoid==0&&ESATakeOverReq==1]
  state OFF
  (default) -> System_Active
  OFF -> System_Active
  System_Active -> OFF

== stateflow chart LACS/AEBsts/AEB_sts ==
  state AEB_ON
    state Default
      entry:AEBsts = 0;
      FCW_Active = 0;
      decel = 0;
    state FCW
      entry:AEBsts = 0;
      FCW_Active = 1;
      decel = 0;
    state Partial_Braking1
      entry:AEBsts = 1;
      FCW_Active = 1;
      decel = CMpa1;
    state Full_Braking
      entry:AEBsts = 3;
      FCW_Active = 1;
      decel = CMpa3;
    state Partial_Braking2
      entry:AEBsts = 2;
      FCW_Active = 1;
      decel = CMpa2;
    (default) -> Default
    Full_Braking -> Default : [stop==1]
    Partial_Braking2 -> Default [order 2] : [stop==1]
    Partial_Braking1 -> Default [order 2] : [stop==1]
    Default -> FCW : [(abs(TTC)<FCWtime)]
    FCW -> Default [order 1] : [abs(TTC)>=1.2*FCWtime]
    FCW -> Partial_Braking1 [order 2] : [(abs(TTC)<PB1time)]
    Partial_Braking1 -> Partial_Braking2 [order 1] : [(abs(TTC)<PB2time)]
    Partial_Braking2 -> Full_Braking [order 1] : [(abs(TTC)<FBtime)]
  (default) -> AEB_ON
  data: TTC input; FCWtime input double; PB1time input double; PB2time input double; FBtime input double; CMpa1 input double; CMpa2 input double; CMpa3 input double; stop input boolean; FCW_Active output; AEBsts output; decel output

== matlab function LACS/CTRL/planning1 ==
  data: vp output; ap output; t input; xr output; yr output; thetar output; kr output
function [vp,ap,xr,yr,thetar,kr] = fcn(t)
    dx=100;
    dy=10;
    T=30;
    xstart=[0,0,0];
    xend=[dx,0,0];
    ystart=[0,0,0];
    yend=[dy,0,0];
    a=zeros(1,6);
    b=zeros(1,6);
    
    a(1)=xstart(1);
    a(2)=xstart(2);
    a(3)=xstart(3)/2;
    A1=[T^3,T^4,T^5;
        3*T^2,4*T^3,5*T^4;
        6*T,12*T^2,20*T^3];
    B1=[xend(1)-a(1)-a(2)*T-a(3)*T^2;
        xend(2)-a(2)-2*a(3)*T;
        xend(3)-2*a(3)];
    xs=inv(A1)*B1;
    a(4)=xs(1);
    a(5)=xs(2);
    a(6)=xs(3);
    b(1)=ystart(1);
    b(2)=ystart(2);
    b(3)=ystart(3)/2;
    A2=[dx^3,dx^4,dx^5;
        3*dx^2,4*dx^3,5*dx^4;
        6*dx,12*dx^2,20*dx^3];
    B2=[yend(1)-b(1)-b(2)*dx-b(3)*dx^2;
        yend(2)-b(2)-2*b(3)*dx;
        yend(3)-2*b(3)];
    ys=inv(A2)*B2;
    b(4)=ys(1);
    b(5)=ys(2);
    b(6)=ys(3);
    xr=a(1)+a(2)*t+a(3)*t^2+a(4)*t^3+a(5)*t^4+a(6)*t^5;
    yr=b(1)+b(2)*xr+b(3)*xr^2+b(4)*xr^3+b(5)*xr^4+b(6)*xr^5;
    xr_dot=a(2)+2*a(3)*t+3*a(4)*t^2+4*a(5)*t^3+5*a(6)*t^4;
    yr_dx=b(2)+2*b(3)*xr+3*b(4)*xr^2+4*b(5)*xr^3+5*b(6)*xr^4;
    yr_dot=yr_dx*xr_dot;
    thetar=atan(yr_dx);
    xr_dot2=2*a(3)+6*a(4)*t+12*a(5)*t^2+20*a(6)*t^3;
    yr_dx2=2*b(3)+6*b(4)*xr+12*b(5)*xr^2+20*b(6)*xr^3;
    yr_dot2=yr_dx2*xr_dot^2+yr_dx*xr_dot2;
    kr=yr_dx2/((1+yr_dx^2)^1.5);
    vp=sqrt(xr_dot^2+yr_dot^2);
    if xr_dot2>=0
        ap=sqrt(xr_dot2^2+yr_dot2^2);
    else
        ap=-sqrt(xr_dot2^2+yr_dot2^2);
    end

== matlab function LACS/ESARegurator_ON/MATLAB Function ==
  data: X_ref input; x_ref output; y_ref output; phi_ref output; x_dot_ref output; y_dot_ref output; phi_dot_ref output; detal_ref output; Y_ref input; Phi_ref input; X_dot_ref input; Y_dot_ref input; Phi_dot_ref input; Detal_ref input; x input; y input
function [x_ref,y_ref,phi_ref,x_dot_ref,y_dot_ref,phi_dot_ref,detal_ref]...
    = get_ref_data(X_ref,Y_ref,Phi_ref,X_dot_ref,Y_dot_ref,Phi_dot_ref,Detal_ref,x,y)
    N=size(X_ref,1);
    min_dis=99999;
    index=1;
    for i=1:N
        cur_dis=sqrt( (x-X_ref(i))^2+(y-Y_ref(i))^2 );
        if cur_dis<min_dis
            index=i;
            min_dis=cur_dis;
        end
    end
    [x_ref,y_ref,phi_ref]=deal(X_ref(index),Y_ref(index),Phi_ref(index));
    [x_dot_ref,y_dot_ref,phi_dot_ref]=deal(X_dot_ref(index),Y_dot_ref(index),Phi_dot_ref(index));
    detal_ref=Detal_ref(index);

== matlab function LACS/ESARegurator_ON/MATLAB Function1 ==
  data: u input; yaw output
function yaw = angle_norm(u)
while u<-2*pi
    u=u+2*pi;
end
while u>2*pi
    u=u-2*pi;
end
yaw = u;
